simulink model "Buck_Boost"  (R2023b)
settings: Solver=ode15s  StartTime=0.0  StopTime=0.025  FixedStep=0.000001  MaxStep=1e-6  RelTol=1e-3
undefined symbols (not defined in the file): C_boost, C_buck, L_boost, L_buck, P_buck_v, P_rec_v, R_buck_load_v, R_rec_load_v, Rl_boost
libraries: simulink x2, slpidlib x1
settings Model: Creator=tudorn  LastModifiedBy=tudorn
settings SolverCC: ZeroCrossAlgorithm=Adaptive
settings DebuggingCC: IgnoredZcDiagnostic=none

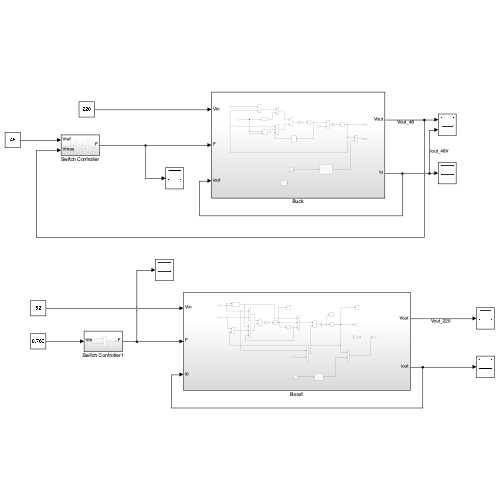
[thumbnail: Simulink's stored preview of the top-level diagram]
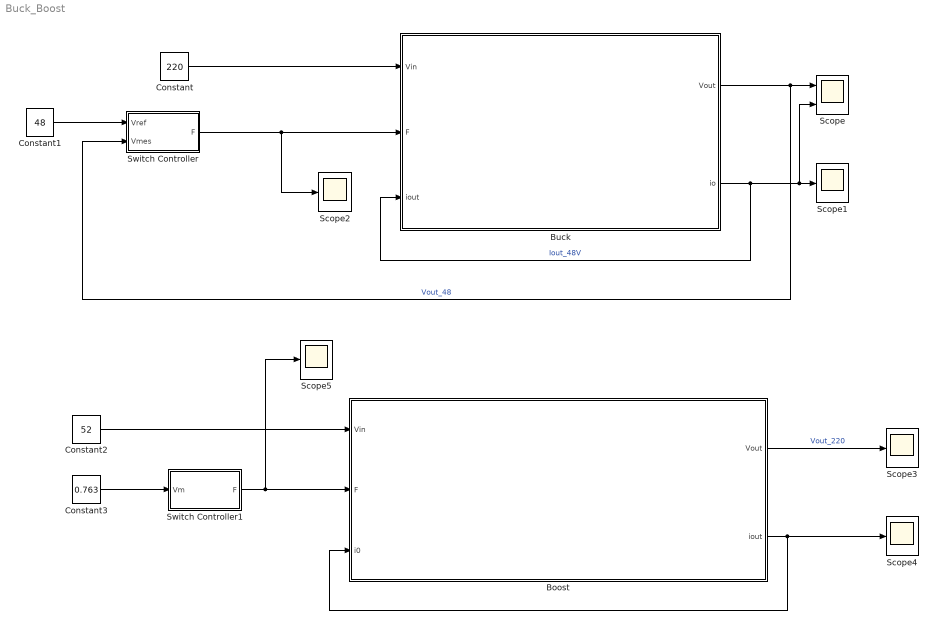
== system Buck_Boost ==
  Boost : Subsystem
  Buck : Subsystem
  Constant : Constant  Value=220
  Constant1 : Constant  Value=48
  Constant2 : Constant  Value=52
  Constant3 : Constant  Value=0.763
  Scope : Scope  NumInputPorts=2
  Scope{1..5} (5 alike) : Scope
  Switch Controller : Subsystem
  Switch Controller1 : Subsystem
  wires:
  Buck/2(io) -> Scope/2, Scope1/1, Buck/3(iout)  "Iout_48V"
  Constant/1 -> Buck/1(Vin)
  Switch Controller/1(F) -> Buck/2(F), Scope2/1
  Constant1/1 -> Switch Controller/1(Vref)
  Buck/1(Vout) -> Switch Controller/2(Vmes), Scope/1  "Vout_48"
  Boost/2(iout) -> Scope4/1, Boost/3(i0)
  Boost/1(Vout) -> Scope3/1  "Vout_220"
  Constant2/1 -> Boost/1(Vin)
  Constant3/1 -> Switch Controller1/1(Vm)
  Switch Controller1/1(F) -> Boost/2(F), Scope5/1

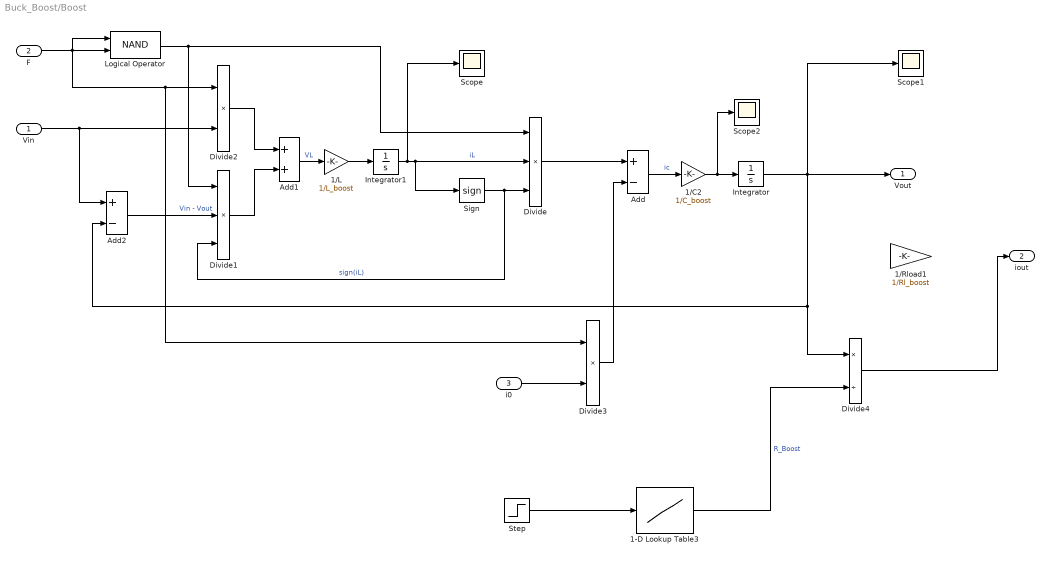
== system Buck_Boost/Boost ==
  Vin : Inport
  F : Inport  Port=2
  i0 : Inport  Port=3
  1-D Lookup Table3 : Lookup_n-D  NumberOfTableDimensions=1  BreakpointsForDimension1=P_rec_v  Table=R_rec_load_v  InternalRulePriority=Speed  RndMeth=Simplest
  1/C2 : Gain  Gain=1/C_boost
  1/L : Gain  Gain=1/L_boost
  1/Rload1 : Gain  Gain=1/Rl_boost
  Add : Sum  Inputs=+-
  Add1 : Sum
  Add2 : Sum  Inputs=+-
  Divide : Product  Inputs=***
  Divide1 : Product  Inputs=***
  Divide2 : Product  Inputs=**
  Divide3 : Product  Inputs=**
  Divide4 : Product  Inputs=*/
  Integrator : Integrator  LimitOutput=on  UpperSaturationLimit=220  LowerSaturationLimit=-220
  Integrator1 : Integrator
  Logical Operator : Logic  Operator=NAND  AllPortsSameDT=off  OutDataTypeStr=boolean
  Scope : Scope
  Scope1 : Scope
  Scope2 : Scope
  Sign : Signum
  Step : Step  Time=0.02  Before=1500  After=2500  SampleTime=0
  Vout : Outport
  iout : Outport  Port=2
  wires:
  Add/1 -> 1/C2/1  "ic"
  Divide/1 -> Add/1
  Sign/1 -> Divide1/3, Divide/3  "sign(iL)"
  1/L/1 -> Integrator1/1
  Integrator1/1 -> Scope/1, Sign/1, Divide/2  "iL"
  Vin/1 -> Add2/1, Divide2/2
  Add2/1 -> Divide1/2  "Vin - Vout"
  F/1 -> Divide2/1, Divide3/1, Logical Operator/1, Logical Operator/2
  Logical Operator/1 -> Divide/1, Divide1/1
  Add1/1 -> 1/L/1  "VL"
  Divide2/1 -> Add1/1
  Divide1/1 -> Add1/2
  i0/1 -> Divide3/2
  Divide3/1 -> Add/2
  Integrator/1 -> Scope1/1, Divide4/1, Add2/2, Vout/1
  1/C2/1 -> Scope2/1, Integrator/1
  1-D Lookup Table3/1 -> Divide4/2  "R_Boost"
  Divide4/1 -> iout/1
  Step/1 -> 1-D Lookup Table3/1

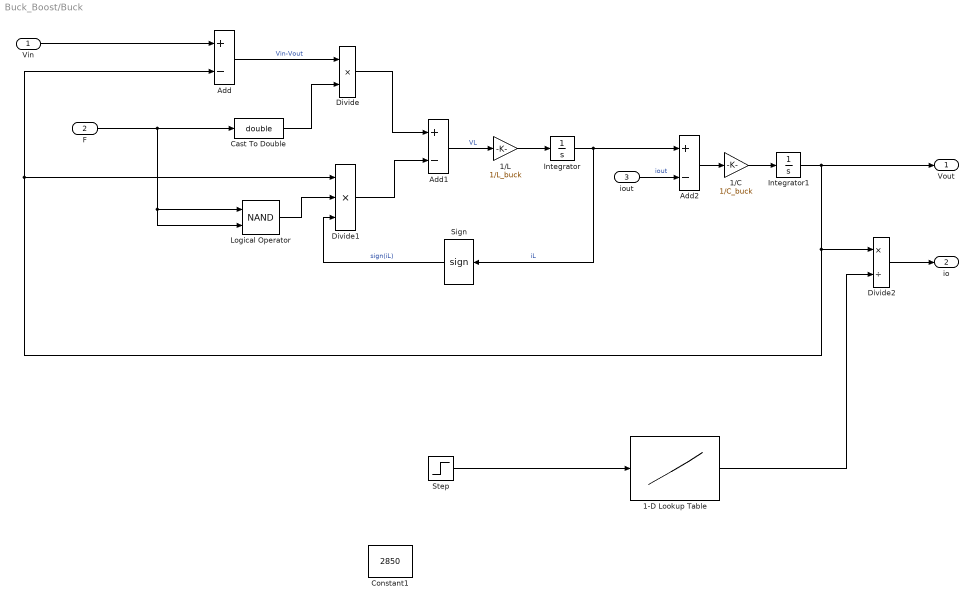
== system Buck_Boost/Buck ==
  Vin : Inport
  F : Inport  Port=2
  iout : Inport  Port=3
  1-D Lookup Table : Lookup_n-D  NumberOfTableDimensions=1  BreakpointsForDimension1=P_buck_v  Table=R_buck_load_v  InternalRulePriority=Speed  RndMeth=Simplest
  1/C : Gain  Gain=1/C_buck
  1/L : Gain  Gain=1/L_buck
  Add : Sum  Inputs=+-
  Add1 : Sum  Inputs=+-
  Add2 : Sum  Inputs=+-
  Cast To Double : DataTypeConversion  OutDataTypeStr=double  SaturateOnIntegerOverflow=off  RndMeth=Floor
  Constant1 : Constant  Value=2850
  Divide : Product  Inputs=**
  Divide1 : Product  Inputs=***
  Divide2 : Product  Inputs=*/
  Integrator : Integrator
  Integrator1 : Integrator
  Logical Operator : Logic  Operator=NAND  AllPortsSameDT=off  OutDataTypeStr=boolean
  Sign : Signum
  Step : Step  Time=0.01  Before=2850  After=4200  SampleTime=0
  Vout : Outport
  io : Outport  Port=2
  wires:
  Vin/1 -> Add/1
  Add/1 -> Divide/1  "Vin-Vout"
  Divide/1 -> Add1/1
  Divide1/1 -> Add1/2
  Add1/1 -> 1/L/1  "VL"
  1/L/1 -> Integrator/1
  Integrator/1 -> Add2/1, Sign/1  "iL"
  Add2/1 -> 1/C/1
  Integrator1/1 -> Divide1/1, Add/2, Divide2/1, Vout/1
  iout/1 -> Add2/2  "iout"
  1/C/1 -> Integrator1/1
  F/1 -> Logical Operator/2, Logical Operator/1, Cast To Double/1
  Sign/1 -> Divide1/3  "sign(iL)"
  Logical Operator/1 -> Divide1/2
  Cast To Double/1 -> Divide/2
  Divide2/1 -> io/1
  1-D Lookup Table/1 -> Divide2/2
  Step/1 -> 1-D Lookup Table/1

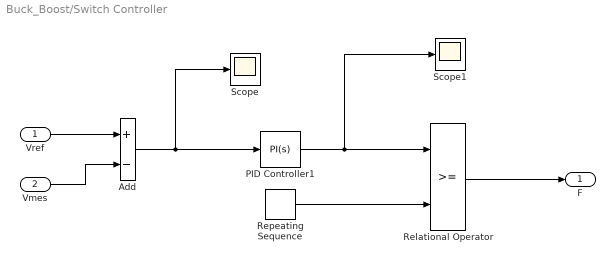
== system Buck_Boost/Switch Controller ==
  Vref : Inport
  Vmes : Inport  Port=2
  Add : Sum  Inputs=+-
  PID Controller1 : slpidlib/PID Controller  Controller=PI  Form=Parallel  TimeDomain=Continuous-time  UseExternalTs=off  SampleTime=-1  IntegratorMethod=Forward Euler  FilterMethod=Forward Euler  ControllerParametersSource=internal  P=0  I=13.2  UseKiTs=off  D=1.7e-5  N=100  UseFilter=on  TunerSelectOption=Transfer Function Based (PID Tuner App)  InitialConditionSource=internal  InitialConditionForIntegrator=0  InitialConditionForFilter=0  DifferentiatorICPrevScaledInput=0  ExternalReset=none  TrackingMode=off  Kt=1  LimitOutput=off  SatLimitsSource=internal  UpperSaturationLimit=inf  LowerSaturationLimit=-inf  LinearizeAsGain=on  AntiWindupMode=none  Kb=1  LimitIntegrator=off  UpperIntegratorSaturationLimit=inf  LowerIntegratorSaturationLimit=-inf  POutMin=[]  POutMax=[]  IOutMin=[]  IOutMax=[]  DOutMin=[]  DOutMax=[]  NOutMin=[]  NOutMax=[]  SumOutMin=[]  SumOutMax=[]  SaturationOutMin=[]  SaturationOutMax=[]  PParamMin=[]  PParamMax=[]  IParamMin=[]  IParamMax=[]  DParamMin=[]  DParamMax=[]  NParamMin=[]  NParamMax=[]  KbParamMin=[]  KbParamMax=[]  KtParamMin=[]  KtParamMax=[]  KbOutMin=[]  KbOutMax=[]  KtOutMin=[]  KtOutMax=[]  IntegratorOutMin=[]  IntegratorOutMax=[]  FilterOutMin=[]  FilterOutMax=[]  SumI1OutMin=[]  SumI1OutMax=[]  SumI2OutMin=[]  SumI2OutMax=[]  SumI3OutMin=[]  SumI3OutMax=[]  SumI4OutMin=[]  SumI4OutMax=[]  SumDOutMin=[]  SumDOutMax=[]  DifferentiatorOutMin=[]  DifferentiatorOutMax=[]  FilterDiffOutCoefMin=[]  FilterDiffOutCoefMax=[]  ReciprocalOutMin=[]  ReciprocalOutMax=[]  SumDenOutMin=[]  SumDenOutMax=[]  SumNumOutMin=[]  SumNumOutMax=[]  DivideOutMin=[]  DivideOutMax=[]  UdiffTsProdOutMin=[]  UdiffTsProdOutMax=[]  NTsProdOutMin=[]  NTsProdOutMax=[]  UintegralTsProdOutMin=[]  UintegralTsProdOutMax=[]  UngainTsProdOutMin=[]  UngainTsProdOutMax=[]  ClampingZeroOutDataTypeStr=Inherit: Inherit via back propagation  ClampingZeroOutMin=[]  ClampingZeroOutMax=[]  FilterDenConstantOutDataTypeStr=Inherit: Inherit via back propagation  FilterDenConstantOutMin=[]  FilterDenConstantOutMax=[]  PCopyOutDataTypeStr=Inherit: Inherit via back propagation  PCopyOutMin=[]  PCopyOutMax=[]  NCopyOutDataTypeStr=Inherit: Inherit via back propagation  NCopyOutMin=[]  NCopyOutMax=[]  IntegratorContinuousStateAttributes=''  IntegratorStateMustResolveToSignalObject=off  IntegratorRTWStateStorageClass=Auto  FilterContinuousStateAttributes=''  FilterStateMustResolveToSignalObject=off  FilterRTWStateStorageClass=Auto  ParallelPVariant=InternalParameters  IdealPVariant=Disabled  IVariant=InternalParameters  DVariant=Disabled  IntegratorVariant=Continuous  SatVariant=Disabled  AWVariant=Passthrough  PCopyVariant=Disabled  TRVariant=Disabled  FdbkBlocksVariant=Forward  IdealPFdbkVariant=Disabled  SatFdbkVariant=Disabled  DerivativeFilterVariant=Disabled  NVariant=Disabled  NCopyVariant=Disabled_SignalSpec  FilterICVariant=Disabled  IntegratorICVariant=InternalICs  ExternalResetVariant=Disabled  TRSumVariant=Passthrough  SumFdbkVariant=Disabled  SumVariant=Sum_PI  TsampFilterVariant=InternalTs  TsampNgainVariant=Passthrough  TsampIntegralVariant=Disabled_SignalSpec  ExternalSaturationOutDataTypeStr=Inherit: Same as second input
  Relational Operator : RelationalOperator  OutDataTypeStr=boolean  RndMeth=Simplest  InputSameDT=off
  Repeating Sequence : simulink/Sources/Repeating Sequence  rep_seq_t=[0, 1e-5, 2e-5]  rep_seq_y=[1, 0, 1]
  Scope : Scope
  Scope1 : Scope
  F : Outport
  wires:
  Relational Operator/1 -> F/1
  Repeating Sequence/1 -> Relational Operator/2
  Vref/1 -> Add/1
  Vmes/1 -> Add/2
  Add/1 -> PID Controller1/1, Scope/1
  PID Controller1/1 -> Scope1/1, Relational Operator/1

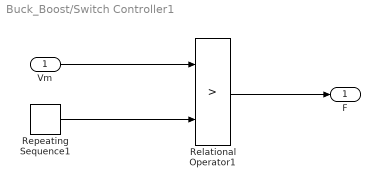
== system Buck_Boost/Switch Controller1 ==
  Vm : Inport
  Relational Operator1 : RelationalOperator  Operator=>  OutDataTypeStr=boolean  RndMeth=Simplest  InputSameDT=off
  Repeating Sequence1 : simulink/Sources/Repeating Sequence  rep_seq_t=[0 0.5 1]/50e3  rep_seq_y=[0 1 0]
  F : Outport
  wires:
  Repeating Sequence1/1 -> Relational Operator1/2
  Relational Operator1/1 -> F/1
  Vm/1 -> Relational Operator1/1
